simulink model "onezonevavdemo"  (R2020a)
settings: Solver=FixedStepAuto  StartTime=0  StopTime=2*24*3600  FixedStep=0.1  RelTol=1e-3
PostLoadFcn:
  | if any(exist('dsrtsu_mdlpostloadfcn', 'file') ~= 0), dsrtsu_mdlpostloadfcn('Execute', bdroot); end
InitFcn:
  | , if any(exist('rtifpga_mdlclblib', 'file') ~= 0), rtifpga_mdlclblib('Init', bdroot); end,
  | , if any(exist('dsmpb_private', 'file') ~= 0), dsmpb_private('dsmpb_mdlclblib', 'Init', bdroot); end,
undefined symbols (not defined in the file): dspaceexample_o_dy2785joocaM
libraries: dsmpblib x7
PreSaveFcn:
  | , if any(exist('dsmpb_private', 'file') ~= 0), dsmpb_private('dsmpb_mdlclblib', 'PreSave', bdroot); end,
CloseFcn:
  | , if any(exist('dsmpb_private', 'file') ~= 0), dsmpb_private('dsmpb_mdlclblib', 'Close', bdroot); end,
settings Model: RTICANMMDATA=struct('GeneralSetupData',struct('modelroot','D:\github\dspace-modelica-example\simulink\onezonevavdemo','generalsettings',struct('filesettings',struct('destfolder',struct('Name','RTICANMM_FILES','Check',1),'buildfolder',struct('Name','.','Check',1),'AbsDestfolder',struct('Name','D:\github\dspace-modelica-example\simulink\onezonevavdemo\RTICANMM_FILES'),'AbsBuildfolder',struct('Name','D:\github\dspace-modelica-example\simulink\onezonevavdemo'))),'options',struct('addpaths',1,'rmpaths',1,'addtrcexclusion',true,'cannavigator',struct('checkmonitoring',0),'show_usrtrc',0,'use_usrtrc',0),'advanced',struct('options',ones(1,100)),'MPSetup',{{}},'RTI',struct('Type','DSRT','Ver','4.3','Date','02-May-2020'),'modelname','onezonevavdemo','block','onezonevavdemo'))  DSRTSU_INTERNAL_RTIFPGA=160  DSMPB_ID_DATA={'100',struct('BlockId','6dd11bb4-ebec-4f08-8ba6-7ddbcbec7d3b','SignalIds',{{'2fb2bb90-4ec6-48ad-8f81-f1d196760c71'}}),'102',struct('BlockId','fcb8ffc9-48d0-43e3-97e6-63db34e8a87a','SignalIds',{{'7405cf0b-34b8-4d18-b681-bf257a32f1fc'}}),'104',struct('BlockId','d3fc6cbc-e5ea-45da-a1ff-e6d33e572c72','SignalIds',{{'ae88789f-7deb-4ded-bc5a-6d8a92166d0d'}}),'199',struct('BlockId','9376efae-c5ba-4aee-a189-875ca35da0c2','SignalIds',{{'13f0521d-e993-4fe3-8f8d-d5fdd3bf7eee'}}),'200',struct('BlockId','0e030ddc-3f5d-48b0-903c-79a8b3e79f79','SignalIds',{{'2dba2b15-4113-4beb-a147-18d9996277b5'}}),'569',struct('BlockId','57008d3f-1417-4acc-b760-eb15ad2b183b','SignalIds',{{'927f367f-c3eb-487d-b017-2942c587586f'}}),'573',struct('BlockId','7d2cb11c-5d6c-46d0-85eb-b23aa6b0ea8f','SignalIds',{{'ea55ac40-3280-4246-b2ec-53e427aefd8d'}})}  Creator=yangyang.fu  LastModifiedBy=yangyang.fu
settings OptimizationCC: BlockReduction=off  ConditionallyExecuteInputs=off  OptimizeBlockIOStorage=off  BufferReuse=off
settings DebuggingCC: TasksWithSamePriorityMsg=none
settings HardwareCC: ProdBitPerPointer=32  ProdBitPerSizeT=32  ProdBitPerPtrDiffT=32  ProdLargestAtomicInteger=Integer  ProdWordSize=32  ProdLongLongMode=on  ProdHWDeviceType=Custom Processor->Custom
settings ModelReferenceCC: EnableParallelModelReferenceBuilds=on
settings SFSimCC: MATLABDynamicMemAlloc=off
settings RTWCC: Description=dSPACE Run-Time Target (for VEOS on Windows and ConfigurationDesk)  SystemTargetFile=dsrt.tlc  GenCodeOnly=on  MakeCommand=make_dsrt  TemplateMakefile=dsrt_default_tmf  RTWVerbose=off  CustomInclude="\"C:\\Program Files\\Dymola 2021\\Source\""
settings STFCustomTargetCC: TargetLangStandard=C99 (ISO)  ParMdlRefBuildCompliant=on  SystemTargetFile=dsrt.tlc
settings GRTTargetCC: CompOptLevelCompliant=off  ConcurrentExecutionCompliant=off  CombineOutputUpdateFcns=off  MatFileLogging=off  CPPClassGenCompliant=off  UseToolchainInfoCompliant=off

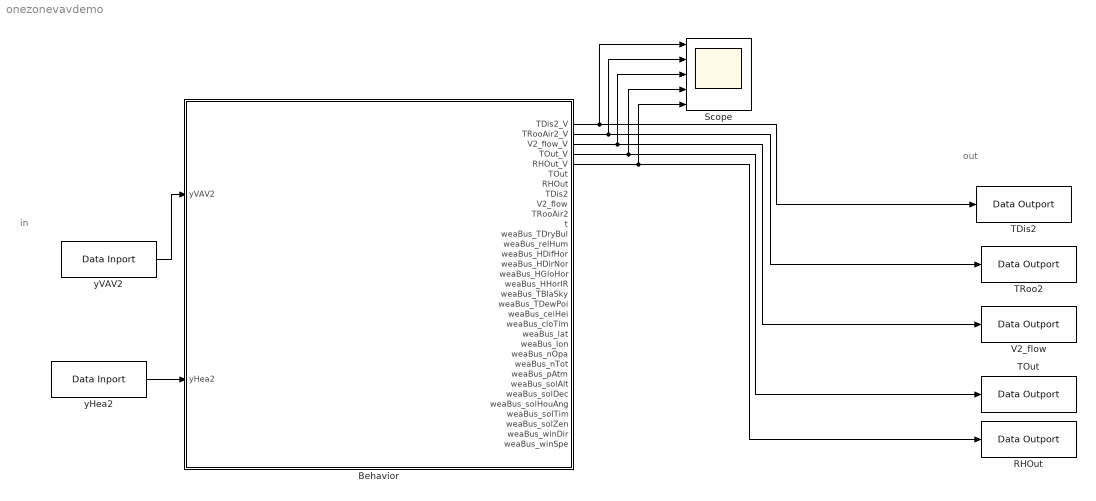
== system onezonevavdemo ==
  note: in
  note: out
  Behavior : Subsystem  Tag=30-Nov-2021 16:26:34#2785  LoadFcn=if exist('newDymolaGui') newDymolaGui('onezonevavdemo/Behavior','PostLoadNew'); else error('Dymola not installed. Must install at least the file newDymolaGui.p'); end;
      mask help:
      | Dymola block.
      | A dymola block allows acausal physical modeling.
      | See Dymola manual for usage.
      settings: CopyFcn=newDymolaGui('30-Nov-2021 16:26:34#2785','Copy');  DeleteFcn=if exist('newDymolaGui') newDymolaGui('onezonevavdemo/Behavior','Delete'); end;  NameChangeFcn=newDymolaGui('30-Nov-2021 16:26:34#2785','Copy');  OpenFcn=newDymolaGui('onezonevavdemo/Behavior','Init');
      mask Display: image(reshape([1;1;1;1;1;1;1;1;1;1;1;1;1;1;1;1;1;1;1;1;1;1;0;0;0;0;0;0;0;0;0;0;1;1;1;1;1;1;1;1;0;1;1;1;1;1;1;1;1;0;1;1;1;1;1;0;0;0;0;0;0;0;1;1;0;0;0;0;0;0;0;1;1;0;0;0;0;0;0;0;1;1;0;0;0;0;0;0;0;1;1;0;0;0;0;0;0;0;1;1;0;0;0;0;0;0;0;1;1;0;0;0;0;0;0;0;1;1;0;0;0;0;0;0;0;1;1;0;0;0;0;0;0;0;1;1;0;0;0;0;0;0;0;1;1;0;0;0;0;0;0;0;1;1;0;0;0;0;0;0;0;1;1;0;0;0;0;0;0;0;1;1;0;0;0;0;0;0;0;1;1;0;0;0;0;0;0;0;1;1;0;0;0;0;0;0;0;1;1;0;0;0;0;0;0;0;1;1;0;0;0;0;0;0;0;1;1;0;0;0;0;0;0;0;1;1;0;0;0;0;0;0;0;1;1;0;0;0;0;0;0;0;1;1;0;0;0;0;0;0;0;1;1;0;0;0;0;0;0;0;1;1;0;0;0;0;0;0;0;1;1;1;1;1;0;1;1;1;1;1;1;1;1;0;1;1;1;1;1;1;1;1;0;0;0;0;0;0;0;0;0;0;1;1;1;1;1;1;1;1;1;1;1;1;1;1;1;1;1;1;1;1;1;1;1;1;1;1;1;1;1;1;1;1;1;1;1;1;1;1;1;1;1;1;1;1;0;0;0;0;0;0;0;0;0;0;1;1;1;1;1;1;1;1;0;1;1;1;1;1;1;1;1;0;1;1;1;1;1;0;0;0;0;0;0;0;1;1;0;0;0;0;0;0;0;1;1;0;0;0;0;0;0;0;1;1;0;0;0;0;0;0;0;1;1;0;0;0;0;0;0;0;1;1;0;0;0;0;0;0;0;1;1;0;0;0;0;0;0;0;1;1;0;0;0;0;0;0;0;1;1;0;0;0;0;0;0;0;1;1;0;0;0;0;0;0;0;1;1;0;0;0;0;0;0;0;1;1;0;0;0;0;0;0;0;1;1;0;0;0;0;0;0;0;1;1;0;0;0;0;0;0;0;1;1;0;0;0;0;0;0;0;1;1;0;0;0;0;0;0;0;1;1;0;0;0;0;0;0;0;1;1;0;0;0;0;0;0;0;1;1;0;0;0;0;0;0;0;1;1;0;0;0;0;0;0;0;1;1;0;0;0;0;0;0;0;1;1;0;0;0;0;0;0;0;1;1;0;0;0;0;0;0;0;1;1;0;0;0;0;0;0;0;1;1;1;1;1;0;1;1;1;1;1;1;1;1;0;1;1;1;1;1;1;1;1;0;0;0;0;0;0;0;0;0;0;1;1;1;1;1;1;1;1;1;1;1;1;1;1;1;1;1;1;1;1;1;1;1;1;1;1;1;1;1;1;1;1;1;1;1;1;1;1;1;1;1;1;1;1;0;0;0;0;0;0;0;0;0;0;1;1;1;1;1;1;1;1;0;1;1;1;1;1;1;1;1;0;1;1;1;1;1;0;0;0;0;0;0;0;1;1;0;0;0;0;0;0;0;1;1;0;1;1;1;1;1;0;1;1;0;1;1;1;1;1;0;1;1;0;1;1;1;1;1;0;1;1;0;1;1;1;1;1;0;1;1;0;1;1;1;1;1;0;1;1;0;1;1;1;1;1;0;1;1;0;1;1;1;1;1;0;1;1;0;1;1;1;1;1;0;1;1;0;1;1;1;1;1;0;1;1;0;1;1;1;1;1;0;1;1;0;1;1;1;1;1;0;1;1;0;1;1;1;1;1;0;1;1;0;1;1;1;1;1;0;1;1;0;1;1;1;1;1;0;1;1;0;1;1;1;1;1;0;1;1;0;1;1;1;1;1;0;1;1;0;1;1;1;1;1;0;1;1;0;1;1;1;1;1;0;1;1;0;1;1;1;1;1;0;1;1;0;1;1;1;1;1;0;1;1;0;0;0;0;0;0;0;1;1;0;0;0;0;0;0;0;1;1;1;1;1;0;1;1;1;1;1;1;1;1;0;1;1;1;1;1;1;1;1;0;0;0;0;0;0;0;0;0;0;1;1;1;1;1;1;1;1;1;1;1;1;1;1;1;1;1;1;1;1;1;1],18,18,3),[.2,.2,.6,.6])
  RHOut : dsmpblib/Data Outport  Priority=-10000
      settings: SourceProductName=dSPACE Model Interface Blockset
  Scope : Scope  NumInputPorts=5
  TDis2 : dsmpblib/Data Outport  Priority=-10000
      settings: SourceProductName=dSPACE Model Interface Blockset
  TOut : dsmpblib/Data Outport  Priority=-10000
      settings: SourceProductName=dSPACE Model Interface Blockset
  TRoo2 : dsmpblib/Data Outport  Priority=-10000
      settings: SourceProductName=dSPACE Model Interface Blockset
  V2_flow : dsmpblib/Data Outport  Priority=-10000
      settings: SourceProductName=dSPACE Model Interface Blockset
  yHea2 : dsmpblib/Data Inport  Priority=10000
      settings: SourceProductName=dSPACE Model Interface Blockset
  yVAV2 : dsmpblib/Data Inport  Priority=10000
      settings: SourceProductName=dSPACE Model Interface Blockset
  wires:
  yVAV2/1 -> Behavior/1(yVAV2)
  Behavior/1(TDis2_V) -> TDis2/1, Scope/1
  Behavior/2(TRooAir2_V) -> Scope/2, TRoo2/1
  Behavior/4(TOut_V) -> Scope/4, TOut/1
  Behavior/5(RHOut_V) -> RHOut/1, Scope/5
  Behavior/3(V2_flow_V) -> Scope/3, V2_flow/1
  yHea2/1 -> Behavior/2(yHea2)

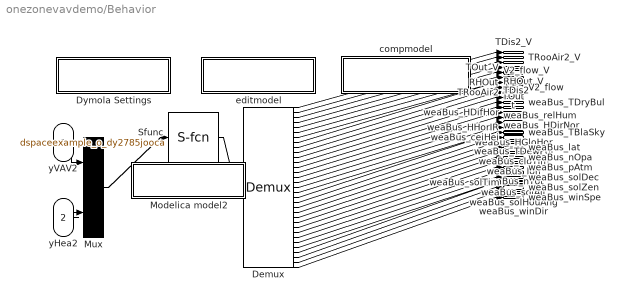
== system onezonevavdemo/Behavior ==
  yVAV2 : Inport
  yHea2 : Inport  Port=2
  Demux : Demux  Outputs=[1;1;1;1;1;1;1;1;1;1;1;1;1;1;1;1;1;1;1;1;1;1;1;1;1;1;1;1;1;1;1;1;1]
  Dymola Settings : Subsystem  mask{ModelName=dSpaceExample.OneZoneVAVUnitConverted, MoFileName=D:/github/dspace-modelica-example/dSpaceExample/OneZoneVAVUnitConverted.mo, dSpace=, BusConnector=[], ResultFile=[], ResultFileOnline=0, ResultDt=[], Libs=:, bigobj=[], ImportFolder=[], guimode=1, ModelName2=[], forRuntime=[], MEXLoad=[], omitDescription=[], ResultName=dspaceexample_o_dy2785jooca}
      mask prompts: ModelName "Name of Dymola model"; MoFileName "File Name (including .mo)"; ResultFile "Create Result"; ResultFileOnline "Load result"; ResultDt "Result min dt"; Libs "Used Libraries"; bigobj "Compiler flag /bigobj"; ImportFolder "Import folder"; guimode "GUI mode flag"; ModelName2 "Model name for import mode"; forRuntime "Runtime export"; MEXLoad "Compiled S-function"; omitDescription "Omit description strings"; ResultName "Name of result file"
      mask Display: disp('Dymola Settings');
  Modelica model2 : Subsystem
      mask Display: disp('Change parameters');
  Mux : Mux  Inputs=[1;1]
  Sfunc : S-Function  Tag=2785jooca  FunctionName=dspaceexample_o_dy2785jooca  Parameters=[dspaceexample_o_dy2785joocaM.pV],[dspaceexample_o_dy2785joocaM.x0V]  PortCounts=[1;1]  SFunctionDeploymentMode=off  EnableBusSupport=off
      mask Display: image(imread('Dymola.bmp'))
  compmodel : Subsystem
      settings: OpenFcn=compileModelica('onezonevavdemo/Behavior');
      mask Display: disp('Compile Modelica model');
  editmodel : Subsystem
      settings: OpenFcn=editModelica('onezonevavdemo/Behavior');
      mask Display: disp('Edit Modelica model');
  TDis2_V : Outport
  TRooAir2_V : Outport  Port=2
  V2_flow_V : Outport  Port=3
  TOut_V : Outport  Port=4
  RHOut_V : Outport  Port=5
  TOut : Outport  Port=6
  RHOut : Outport  Port=7
  TDis2 : Outport  Port=8
  V2_flow : Outport  Port=9
  TRooAir2 : Outport  Port=10
  t : Outport  Port=11
  weaBus_TDryBul : Outport  Port=12
  weaBus_relHum : Outport  Port=13
  weaBus_HDifHor : Outport  Port=14
  weaBus_HDirNor : Outport  Port=15
  weaBus_HGloHor : Outport  Port=16
  weaBus_HHorIR : Outport  Port=17
  weaBus_TBlaSky : Outport  Port=18
  weaBus_TDewPoi : Outport  Port=19
  weaBus_ceiHei : Outport  Port=20
  weaBus_cloTim : Outport  Port=21
  weaBus_lat : Outport  Port=22
  weaBus_lon : Outport  Port=23
  weaBus_nOpa : Outport  Port=24
  weaBus_nTot : Outport  Port=25
  weaBus_pAtm : Outport  Port=26
  weaBus_solAlt : Outport  Port=27
  weaBus_solDec : Outport  Port=28
  weaBus_solHouAng : Outport  Port=29
  weaBus_solTim : Outport  Port=30
  weaBus_solZen : Outport  Port=31
  weaBus_winDir : Outport  Port=32
  weaBus_winSpe : Outport  Port=33
  wires:
  Sfunc/1 -> Demux/1
  Demux/1 -> TDis2_V/1
  Demux/2 -> TRooAir2_V/1
  Demux/3 -> V2_flow_V/1
  Demux/4 -> TOut_V/1
  Demux/5 -> RHOut_V/1
  Demux/6 -> TOut/1
  Demux/7 -> RHOut/1
  Demux/8 -> TDis2/1
  Demux/9 -> V2_flow/1
  Demux/10 -> TRooAir2/1
  Demux/11 -> t/1
  Demux/12 -> weaBus_TDryBul/1
  Demux/13 -> weaBus_relHum/1
  Demux/14 -> weaBus_HDifHor/1
  Demux/15 -> weaBus_HDirNor/1
  Demux/16 -> weaBus_HGloHor/1
  Demux/17 -> weaBus_HHorIR/1
  Demux/18 -> weaBus_TBlaSky/1
  Demux/19 -> weaBus_TDewPoi/1
  Demux/20 -> weaBus_ceiHei/1
  Demux/21 -> weaBus_cloTim/1
  Demux/22 -> weaBus_lat/1
  Demux/23 -> weaBus_lon/1
  Demux/24 -> weaBus_nOpa/1
  Demux/25 -> weaBus_nTot/1
  Demux/26 -> weaBus_pAtm/1
  Demux/27 -> weaBus_solAlt/1
  Demux/28 -> weaBus_solDec/1
  Demux/29 -> weaBus_solHouAng/1
  Demux/30 -> weaBus_solTim/1
  Demux/31 -> weaBus_solZen/1
  Demux/32 -> weaBus_winDir/1
  Demux/33 -> weaBus_winSpe/1
  Mux/1 -> Sfunc/1
  yVAV2/1 -> Mux/1
  yHea2/1 -> Mux/2

== system onezonevavdemo/Behavior/Dymola Settings ==

== system onezonevavdemo/Behavior/Modelica model2 ==

== system onezonevavdemo/Behavior/compmodel ==

== system onezonevavdemo/Behavior/editmodel ==
